simulink model "Newton_Euler_Rotational_Motion"  (R2018a)
settings: Solver=VariableStepAuto  StartTime=0.0  StopTime=10.0  RelTol=1e-3
settings Model: Creator=Ibrahim  LastModifiedBy=Ibrahim

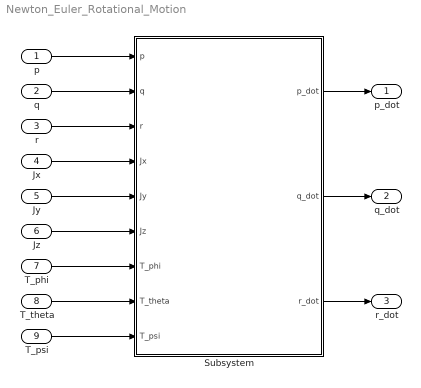
== system Newton_Euler_Rotational_Motion ==
  p : Inport
  q : Inport  Port=2
  r : Inport  Port=3
  Jx : Inport  Port=4
  Jy : Inport  Port=5
  Jz : Inport  Port=6
  T_phi : Inport  Port=7
  T_theta : Inport  Port=8
  T_psi : Inport  Port=9
  Subsystem : Subsystem
  p_dot : Outport
  q_dot : Outport  Port=2
  r_dot : Outport  Port=3
  wires:
  p/1 -> Subsystem/1(p)
  q/1 -> Subsystem/2(q)
  r/1 -> Subsystem/3(r)
  Jx/1 -> Subsystem/4(Jx)
  Jy/1 -> Subsystem/5(Jy)
  Jz/1 -> Subsystem/6(Jz)
  T_phi/1 -> Subsystem/7(T_phi)
  T_theta/1 -> Subsystem/8(T_theta)
  T_psi/1 -> Subsystem/9(T_psi)
  Subsystem/1(p_dot) -> p_dot/1
  Subsystem/2(q_dot) -> q_dot/1
  Subsystem/3(r_dot) -> r_dot/1

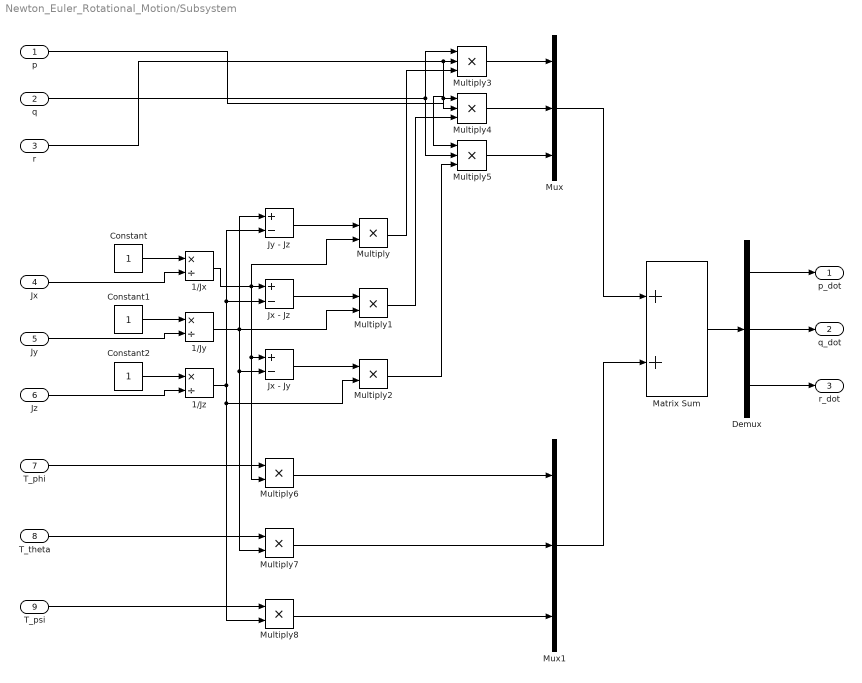
== system Newton_Euler_Rotational_Motion/Subsystem ==
  p : Inport
  q : Inport  Port=2
  r : Inport  Port=3
  Jx : Inport  Port=4
  Jy : Inport  Port=5
  Jz : Inport  Port=6
  T_phi : Inport  Port=7
  T_theta : Inport  Port=8
  T_psi : Inport  Port=9
  1/Jx : Product  Inputs=*/
  1/Jy : Product  Inputs=*/
  1/Jz : Product  Inputs=*/
  Constant : Constant
  Constant1 : Constant
  Constant2 : Constant
  Demux : Demux  Outputs=3
  Jx - Jy : Sum  Inputs=+-
  Jx - Jz : Sum  Inputs=+-
  Jy - Jz : Sum  Inputs=+-
  Matrix Sum : Sum
  Multiply{,1..2,6..8} (6 alike) : Product
  Multiply3 : Product  Inputs=3
  Multiply4 : Product  Inputs=3
  Multiply5 : Product  Inputs=3
  Mux : Mux  Inputs=3
  Mux1 : Mux  Inputs=3
  p_dot : Outport
  q_dot : Outport  Port=2
  r_dot : Outport  Port=3
  wires:
  T_psi/1 -> Multiply8/1
  Multiply4/1 -> Mux/2
  Multiply8/1 -> Mux1/3
  1/Jz/1 -> Multiply2/2, Multiply8/2, Jx - Jz/2, Jy - Jz/2
  1/Jy/1 -> Jx - Jy/2, Multiply7/2, Jy - Jz/1, Multiply1/2
  r/1 -> Multiply4/2, Multiply3/2
  Multiply3/1 -> Mux/1
  q/1 -> Multiply3/1, Multiply5/2
  Jx - Jz/1 -> Multiply1/1
  Jy - Jz/1 -> Multiply/1
  T_theta/1 -> Multiply7/1
  Multiply/1 -> Multiply3/3
  Demux/1 -> p_dot/1
  Constant2/1 -> 1/Jz/1
  Multiply7/1 -> Mux1/2
  Multiply6/1 -> Mux1/1
  Jy/1 -> 1/Jy/2
  Jx/1 -> 1/Jx/2
  p/1 -> Multiply5/1, Multiply4/1
  1/Jx/1 -> Jx - Jy/1, Multiply6/2, Jx - Jz/1, Multiply/2
  Jx - Jy/1 -> Multiply2/1
  Constant/1 -> 1/Jx/1
  Jz/1 -> 1/Jz/2
  Demux/3 -> r_dot/1
  Mux/1 -> Matrix Sum/1
  Mux1/1 -> Matrix Sum/2
  T_phi/1 -> Multiply6/1
  Matrix Sum/1 -> Demux/1
  Constant1/1 -> 1/Jy/1
  Multiply5/1 -> Mux/3
  Multiply1/1 -> Multiply4/3
  Demux/2 -> q_dot/1
  Multiply2/1 -> Multiply5/3
